simulink model "GeneratedModelTest"  (R2014b)
settings: Solver=ode3  StartTime=0.0  StopTime=7  FixedStep=0.045  RelTol=1e-9
settings Model: Creator=levente.nagy960115  LastModifiedBy=levente.nagy960115

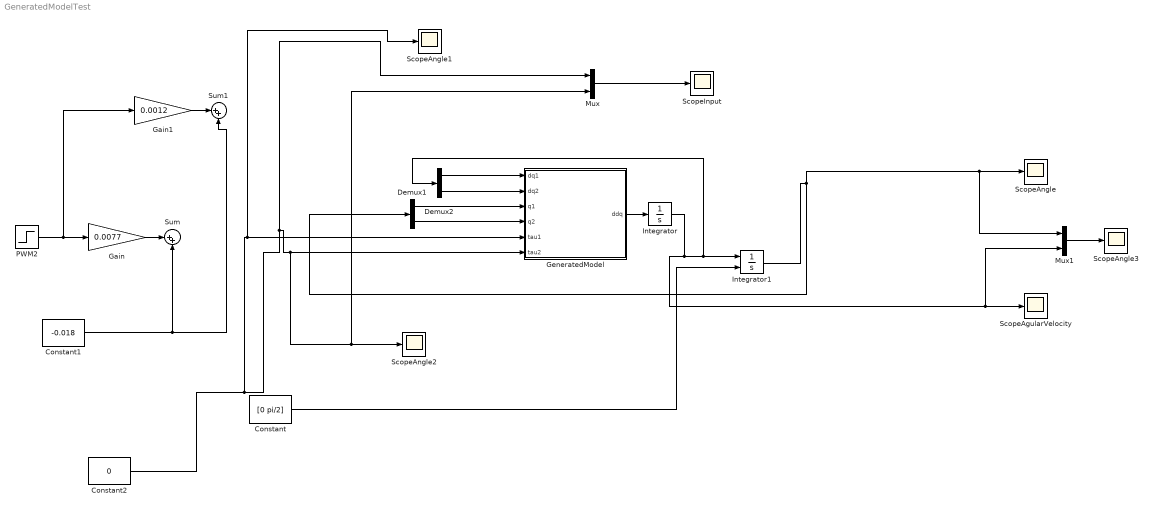
== system GeneratedModelTest ==
  Constant : Constant  Value=[0 pi/2]
  Constant1 : Constant  Value=-0.018
  Constant2 : Constant  Value=0
  Demux1 : Demux  Outputs=2
  Demux2 : Demux  Outputs=2
  Gain : Gain  Gain=0.0077
  Gain1 : Gain  Gain=0.0012
  GeneratedModel : MATLAB Function  TreatAsAtomicUnit=on
  Integrator : Integrator  InitialCondition=[0 0]
  Integrator1 : Integrator  InitialConditionSource=external  InitialCondition=[0 pi-0.1 0.1]
  Mux : Mux  Inputs=2
  Mux1 : Mux  Inputs=2
  PWM2 : Step  Time=0  After=0
  ScopeAgularVelocity : Scope
      settings: TimeRange=10  YMin=-40  YMax=30  SaveName=jointVelocity
  ScopeAngle{,1..3} (4 alike) : Scope
      ScopeAngle settings: TimeRange=16  YMax=2  SaveName=jointAngles
      ScopeAngle1 settings: TimeRange=10  YMin=0  SaveName=jointAngles1
      ScopeAngle2 settings: TimeRange=10  YMin=0  SaveName=jointAngles2
      ScopeAngle3 settings: TimeRange=10  YMin=0  SaveName=SimulationStates
  ScopeInput : Scope
      settings: TimeRange=10  YMin=0  SaveName=jointInput
  Sum : Sum  Inputs=|++
  Sum1 : Sum  Inputs=|++
  wires:
  GeneratedModel/1(ddq) -> Integrator/1
  Integrator/1 -> Mux1/2, ScopeAgularVelocity/1, Demux2/1, Integrator1/1
  Integrator1/1 -> Demux1/1, Mux1/1, ScopeAngle/1
  Constant/1 -> Integrator1/2
  Demux2/1 -> GeneratedModel/1(dq1)
  Demux2/2 -> GeneratedModel/2(dq2)
  Demux1/2 -> GeneratedModel/4(q2)
  Mux/1 -> ScopeInput/1
  Mux1/1 -> ScopeAngle3/1
  PWM2/1 -> Gain1/1, Gain/1
  Demux1/1 -> GeneratedModel/3(q1)
  Gain/1 -> Sum/1
  Constant1/1 -> Sum1/2, Sum/2
  Gain1/1 -> Sum1/1
  Constant2/1 -> ScopeAngle1/1, GeneratedModel/5(tau1), Mux/1, Mux/2, ScopeAngle2/1, GeneratedModel/6(tau2)

== matlab function GeneratedModelTest/GeneratedModel ==
  data: dq1 input; ddq output; dq2 input; q1 input; q2 input; tau1 input; tau2 input
function ddq = GeneratedModel(dq1,dq2,q1,q2,tau1,tau2)
%#codegen

%    This function was generated by the Symbolic Math Toolbox version 6.1.
%    06-Jan-2017 15:50:02

t2 = cos(q2);
t3 = t2.*1.621007635477227e20;
t4 = t2.^2;
t5 = t4.*4.324164689001009e19;
t6 = t3+t5+1.714360266165995e20;
t7 = 1.0./t6;
t8 = sin(q2);
t9 = q2.*2.0;
t10 = sin(t9);
ddq = [-dq1.*(t7.*1.106804644422573e22-dq2.*t7.*(t8.*4.265809567045334e19+t10.*1.137938076052897e19).*(1.9e1./5.0))+t7.*tau1.*4.611686018427388e22+t7.*sin(q1).*(t2.*1.48e3+3.173e3).*5.655079980096584e18;dq2.*(-6.785699139064422)+tau2.*4.241061961915264e1-dq1.^2.*(t8.*7.453666398066076e-2+t10.*1.988323826286102e-2)+t8.*cos(q1).*7.696891301581916];
